simulink model "q_3dgyro_quick_start"  (R2024b)
settings: Solver=ode1  StartTime=0.0  StopTime=inf  FixedStep=0.002  RelTol=1e-3  EnableMultiTasking=on
PostLoadFcn:
  | qc_set_target_type(getConfigSet(bdroot, 'QUARC Default Target Configuration'));
undefined symbols (not defined in the file): HIL, qc_get_step_size
libraries: quarc_library x4, simulink x2
settings Model: SimulationMode=external  ExtModeTrigDuration=5000  Creator=pmartin  LastModifiedBy=dmfde
settings SolverCC: AlgebraicLoopSolver=TrustRegion  PositivePriorityOrder=on
settings DataIOCC: Decimation=10  LimitDataPoints=on  MaxDataPoints=100000  SaveFormat=Array  SignalLoggingSaveFormat=ModelDataLogs  ReturnWorkspaceOutputs=off
settings OptimizationCC: ExpressionDepthLimit=2147483647  InitFltsAndDblsToZero=on
settings DebuggingCC: SaveWithParameterizedLinksMsg=none  UnderspecifiedInitializationDetection=Classic  MergeDetectMultiDrivingBlocksExec=none  SolverPrmCheckMsg=warning  MultiTaskDSMMsg=warning  MultiTaskCondExecSysMsg=none  FcnCallInpInsideContextMsg=warning  UnconnectedInputMsg=warning  UnconnectedOutputMsg=warning  UnconnectedLineMsg=warning  StateNameClashWarn=warning  SFUnexpectedBacktrackingDiag=warning  SFNoUnconditionalDefaultTransitionDiag=warning  SFExecutionAtInitializationDiag=none  ArithmeticOperatorsInVariantConditions=warning
settings ModelReferenceCC: PropagateSignalLabelsOutOfModel=off
settings SFSimCC: SimUseLocalCustomCode=off  CustomCodeUndefinedFunction=UseInterfaceOnly
settings RTWCC: Description=QUARC Win64 Target Using Toolchain  SystemTargetFile=quarc_win64.tlc  TemplateMakefile=quarc_default_tmf  RTWUseLocalCustomCode=off  Toolchain=QUARC win64 | nmake (64-bit Windows)  BuildConfiguration=Faster Runs  GPUComputeCapability=3.5
settings CodeAppCC: StateflowObjectComments=on
settings STFCustomTargetCC: ConcurrentExecutionCompliant=on  GRTInterface=on  UseToolchainInfoCompliant=on  SystemTargetFile=quarc_win64.tlc
settings GRTTargetCC: TargetLangStandard=C89/C90 (ANSI)  ParMdlRefBuildCompliant=off  CompOptLevelCompliant=off  CombineOutputUpdateFcns=off  MatFileLogging=off  CPPClassGenCompliant=off  GRTInterface=on  ExtMode=on  ExtModeStaticAllocSize=10000000  ExtModeMexFile=quarc_comm
settings ConfigComp: CovMetricSettings=dw  CovSaveCumulativeToWorkspaceVar=on  CovSaveSingleToWorkspaceVar=on  CovExternalEMLEnable=off

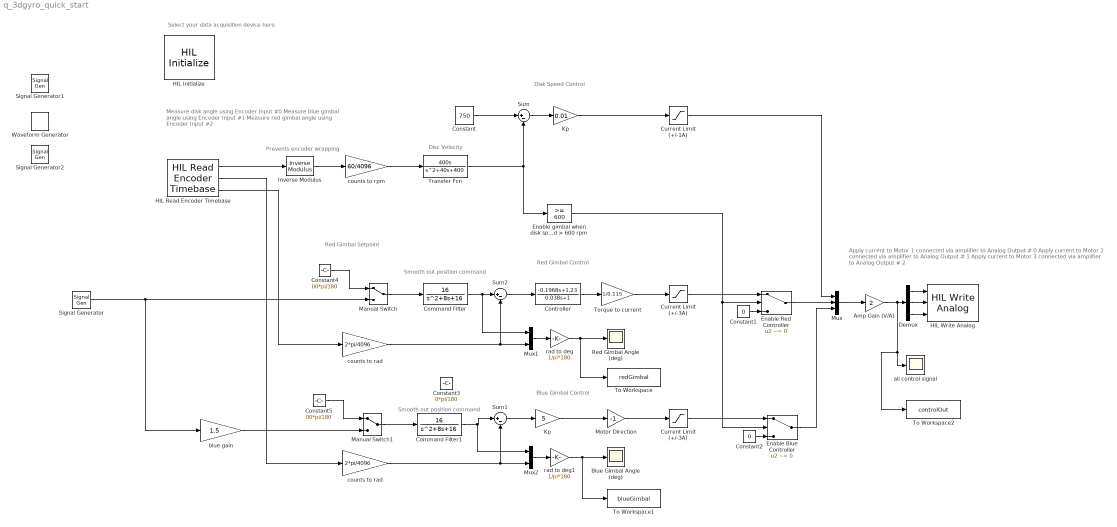
== system q_3dgyro_quick_start ==
  note: Smooth out position command
  note: Disc Velocity
  note: Prevents encoder wrapping
  note: Select your data acquisition device here.
  note: Disk Speed Control
  note: Red Gimbal Control
  note: Blue Gimbal Control
  note: Red Gimbal Setpoint
  note: Measure disk angle using Encoder Input  #0
      | Measure blue gimbal angle using Encoder Input #1
      | Measure red gimbal angle using Encoder Input #2
  note: Apply current to Motor 1 connected via amplifier to Analog Output # 0
      | Apply current to Motor 2 connected via amplifier to Analog Output # 1
      | Apply current to Motor 3 connected via amplifier to Analog Output # 2
  note: Smooth out position command
  Amp Gain (V/A) : Gain  Gain=2
  Blue Gimbal Angle (deg) : Scope
  Command Filter : TransferFcn  Numerator=[16]  Denominator=[1 8 16]
  Command Filter1 : TransferFcn  Numerator=[16]  Denominator=[1 8 16]
  Constant : Constant  Value=750
  Constant1 : Constant  Value=0
  Constant2 : Constant  Value=0
  Constant3 : Constant  Value=0*pi/180
  Constant4 : Constant  Value=00*pi/180
  Constant5 : Constant  Value=00*pi/180
  Controller : TransferFcn  Numerator=[-0.1968 1.23]  Denominator=[0.038 1]
  Current Limit (+/-1A) : Saturate  UpperLimit=1  LowerLimit=-1
  Current Limit (+/-3A) : Saturate  UpperLimit=3  LowerLimit=-3
  "Current Limit (+/-3A) " : Saturate  UpperLimit=3  LowerLimit=-3
  Demux : Demux  Outputs=3
  Enable Blue Controller : Switch  Criteria=u2 ~= 0  SaturateOnIntegerOverflow=off  InputSameDT=off
  Enable Red Controller : Switch  Criteria=u2 ~= 0  SaturateOnIntegerOverflow=off  InputSameDT=off
  Enable gimbal when disk speed > 600 rpm : simulink/Logic and Bit Operations/Compare To Constant  relop=>=  const=600  OutDataTypeStr=boolean
  HIL Initialize : quarc_library/Data Acquisition/Generic/Configuration/HIL Initialize  Priority=-99  object_name=HIL-1  board_type=q8_usb  board_number=0  board_options=update_rate=normal;decimation=1  exclusive=off  active=off  hardware_clocks=[0:2]  clock_modes=[]  initial_clock_frequencies=[]  set_clock_params_at_start=off  set_clock_params_at_switch_in=off  set_clock_frequencies_at_start=off  set_clock_frequencies_at_switch_in=off  analog_input_channels=[0:7]  analog_input_configurations=[]  analog_input_maximums=10  analog_input_minimums=-10  set_analog_input_params_at_start=on  set_analog_input_params_at_switch_in=off  analog_output_channels=[0:7]  analog_output_maximums=10  analog_output_minimums=-10  initial_analog_outputs=[0]  final_analog_outputs=[0]  watchdog_analog_outputs=0  set_analog_output_params_at_start=on  set_analog_output_params_at_switch_in=off  set_analog_outputs_at_start=on  set_analog_outputs_at_switch_in=off  set_analog_outputs_at_terminate=on  set_analog_outputs_at_switch_out=off  set_analog_outputs_on_watchdog=off  digital_input_channels=[]  digital_output_channels=[0:4]  digital_output_configuration=[]  initial_digital_outputs=[0 0 0 0 1]  final_digital_outputs=[1 1 1 1 0]  watchdog_digital_outputs=[1 1 1 1 0]  set_digital_output_params_at_start=off  set_digital_output_params_at_switch_in=off  set_digital_outputs_at_start=on  set_digital_outputs_at_switch_in=off  set_digital_outputs_at_terminate=on  set_digital_outputs_at_switch_out=off  set_digital_outputs_on_watchdog=off  encoder_channels=[0:7]  quadrature=[4]  encoder_filter_frequency=[]  initial_encoder_counts=[0]  set_encoder_params_at_start=on  set_encoder_params_at_switch_in=off  set_encoder_counts_at_start=on  set_encoder_counts_at_switch_in=off  pwm_channels=[0:7]  pwm_modes=0  pwm_frequency=99.532799999999995e6/4095  pwm_configuration=[0]  pwm_alignment=[0]  pwm_polarity=[1]  pwm_leading_deadband=[0]  pwm_trailing_deadband=[0]  initial_pwm_outputs=[0]  final_pwm_outputs=[0]  watchdog_pwm_outputs=[0]  set_pwm_params_at_start=on  set_pwm_params_at_switch_in=off  set_pwm_outputs_at_start=on  set_pwm_outputs_at_switch_in=off  set_pwm_outputs_at_terminate=on  set_pwm_outputs_at_switch_out=off  set_pwm_outputs_on_watchdog=off  other_output_channels=[]  initial_other_outputs=[]  final_other_outputs=[]  watchdog_other_outputs=[]  set_other_outputs_at_start=off  set_other_outputs_at_switch_in=off  set_other_outputs_at_terminate=off  set_other_outputs_at_switch_out=off  set_other_outputs_on_watchdog=off
  HIL Read Encoder Timebase : quarc_library/Data Acquisition/Generic/Timebases/HIL Read Encoder Timebase  object_name=HIL-1  clock=0  channels=0:2  active=on  vector_output=off  data_type_mode=Inherit via back propagation  data_type=double  overflow_mode=Error on overflow  samples_in_buffer=max(ceil(1/qc_get_step_size), 1)
  HIL Write Analog : quarc_library/Data Acquisition/Generic/Immediate I//O/HIL Write Analog  object_name=HIL-1  channels=0:2  sample_time=-1  active=off  vector_input=off
  Inverse Modulus : quarc_library/Discontinuities/Inverse Modulus  modulus=16777215  output_derivative=off  output_revolutions=off  max_x=Inf  min_x=-Inf
  Kp : Gain  Gain=0.01
  "Kp " : Gain  Gain=5
  Manual Switch : ManualSwitch
  Manual Switch1 : ManualSwitch
  Motor Direction : Gain  Gain=-1
  Mux : Mux  Inputs=3
  Mux1 : Mux  Inputs=2
  Mux2 : Mux  Inputs=2
  Red Gimbal Angle (deg) : Scope
  Signal Generator : SignalGenerator  Amplitude=20/180*pi  Frequency=0.2
  Signal Generator1 : SignalGenerator  WaveForm=square  Amplitude=10/180*pi  Frequency=0.2
  Signal Generator2 : SignalGenerator  Amplitude=10/180*pi  Frequency=0.2
  Sum : Sum  Inputs=|+-
  Sum1 : Sum  Inputs=|+-
  Sum2 : Sum  Inputs=|+-
  To Workspace : ToWorkspace  VariableName=redGimbal  SampleTime=-1
      settings: Save2DSignal=2-D array (concatenate along first dimension)
  To Workspace1 : ToWorkspace  VariableName=blueGimbal  SampleTime=-1
      settings: Save2DSignal=2-D array (concatenate along first dimension)
  To Workspace2 : ToWorkspace  VariableName=controlOut  SampleTime=-1
      settings: Save2DSignal=2-D array (concatenate along first dimension)
  Torque to current : Gain  Gain=1/0.115
  Transfer Fcn : TransferFcn  Numerator=[400 0]  Denominator=[1 40 400]
  Waveform Generator : simulink/Sources/Waveform Generator  OutMin=[]  OutMax=[]  OutDataTypeStr=double  SelectedSignal=1  Signals=sin(20*pi/180,.2,0)  BlockNames=MultiportSwitch_212bafd19241474  SampleTime=0.1
  all control signal : Scope
  blue gain : Gain  Gain=1.5
  counts to rad : Gain  Gain=2*pi/4096
  "counts to rad " : Gain  Gain=2*pi/4096
  counts to rpm : Gain  Gain=60/4096
  rad to deg : Gain  Gain=1/pi*180
  rad to deg1 : Gain  Gain=1/pi*180
  wires:
  HIL Read Encoder Timebase/1 -> Inverse Modulus/1
  Inverse Modulus/1 -> counts to rpm/1
  counts to rpm/1 -> Transfer Fcn/1
  Constant/1 -> Sum/1
  Transfer Fcn/1 -> Enable gimbal when disk speed > 600 rpm/1, Sum/2
  Sum/1 -> Kp/1
  Kp/1 -> Current Limit (+/-1A)/1
  Constant1/1 -> Enable Red Controller/3
  Enable gimbal when disk speed > 600 rpm/1 -> Enable Blue Controller/2, Enable Red Controller/2
  Constant2/1 -> Enable Blue Controller/3
  Sum1/1 -> "Kp "/1
  "Kp "/1 -> Motor Direction/1
  Motor Direction/1 -> "Current Limit (+/-3A) "/1
  "Current Limit (+/-3A) "/1 -> Enable Blue Controller/1
  "counts to rad "/1 -> Mux2/2, Sum1/2
  HIL Read Encoder Timebase/2 -> "counts to rad "/1
  Constant4/1 -> Manual Switch/1
  Manual Switch/1 -> Command Filter/1
  Command Filter/1 -> Mux1/1, Sum2/1
  HIL Read Encoder Timebase/3 -> counts to rad/1
  Sum2/1 -> Controller/1
  Controller/1 -> Torque to current/1
  Torque to current/1 -> Current Limit (+/-3A)/1
  counts to rad/1 -> Mux1/2, Sum2/2
  Current Limit (+/-3A)/1 -> Enable Red Controller/1
  Mux/1 -> Amp Gain (V/A)/1
  Enable Red Controller/1 -> Mux/2
  Enable Blue Controller/1 -> Mux/3
  Current Limit (+/-1A)/1 -> Mux/1
  Amp Gain (V/A)/1 -> To Workspace2/1, all control signal/1, Demux/1
  Demux/1 -> HIL Write Analog/1
  Demux/2 -> HIL Write Analog/2
  Demux/3 -> HIL Write Analog/3
  rad to deg/1 -> To Workspace/1, Red Gimbal Angle (deg)/1
  rad to deg1/1 -> To Workspace1/1, Blue Gimbal Angle (deg)/1
  Mux1/1 -> rad to deg/1
  Mux2/1 -> rad to deg1/1
  Signal Generator/1 -> Manual Switch/2, blue gain/1
  Manual Switch1/1 -> Command Filter1/1
  Constant5/1 -> Manual Switch1/1
  Command Filter1/1 -> Mux2/1, Sum1/1
  blue gain/1 -> Manual Switch1/2
